simulink model "TST_RmtAPP_Kickdown"  (R2016b)
settings: Solver=FixedStepDiscrete  StartTime=0.0  StopTime=simTime  FixedStep=sampleTime  RelTol=1e-3
values from neighbouring files (symbols this model uses):
  testCase = 1    [initTST_RmtAPP_Kickdown_001.m]    (also in initTST_RmtAPP_Kickdown_002.m = 2; initTST_RmtAPP_Kickdown_003.m = 3)
libraries: simulink x7, UnitTest_Lib x3
settings Model: Creator=bianxuyin  LastModifiedBy=bianxuyin
settings DebuggingCC: SignalRangeChecking=error

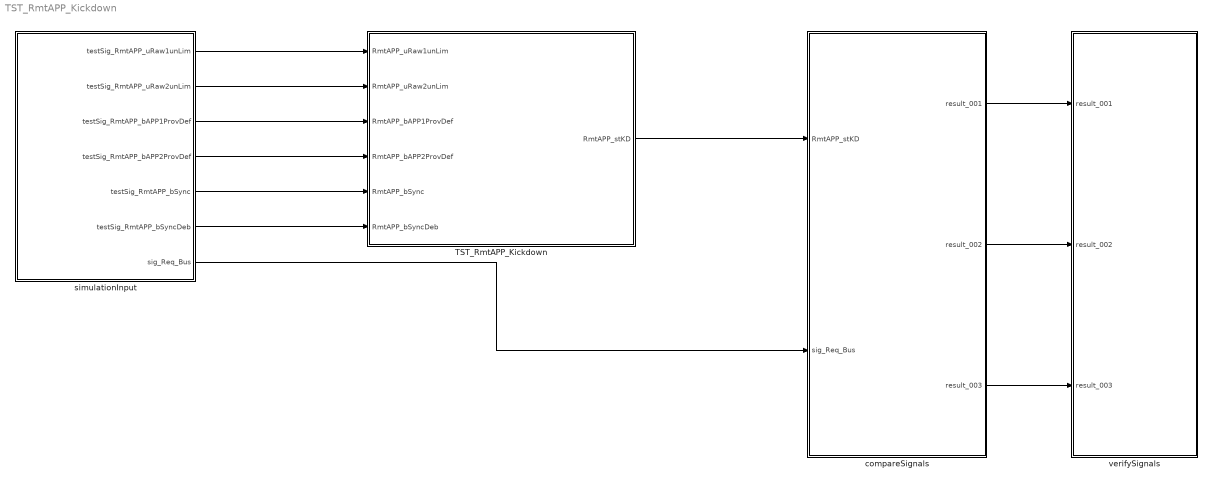
== system TST_RmtAPP_Kickdown ==
  TST_RmtAPP_Kickdown : Subsystem
  compareSignals : Subsystem
  simulationInput : Subsystem
  verifySignals : Subsystem
  wires:
  simulationInput/1(testSig_RmtAPP_uRaw1unLim) -> TST_RmtAPP_Kickdown/1(RmtAPP_uRaw1unLim)
  simulationInput/2(testSig_RmtAPP_uRaw2unLim) -> TST_RmtAPP_Kickdown/2(RmtAPP_uRaw2unLim)
  simulationInput/3(testSig_RmtAPP_bAPP1ProvDef) -> TST_RmtAPP_Kickdown/3(RmtAPP_bAPP1ProvDef)
  simulationInput/4(testSig_RmtAPP_bAPP2ProvDef) -> TST_RmtAPP_Kickdown/4(RmtAPP_bAPP2ProvDef)
  simulationInput/5(testSig_RmtAPP_bSync) -> TST_RmtAPP_Kickdown/5(RmtAPP_bSync)
  simulationInput/6(testSig_RmtAPP_bSyncDeb) -> TST_RmtAPP_Kickdown/6(RmtAPP_bSyncDeb)
  TST_RmtAPP_Kickdown/1(RmtAPP_stKD) -> compareSignals/1(RmtAPP_stKD)
  simulationInput/7(sig_Req_Bus) -> compareSignals/2(sig_Req_Bus)
  compareSignals/1(result_001) -> verifySignals/1(result_001)
  compareSignals/2(result_002) -> verifySignals/2(result_002)
  compareSignals/3(result_003) -> verifySignals/3(result_003)

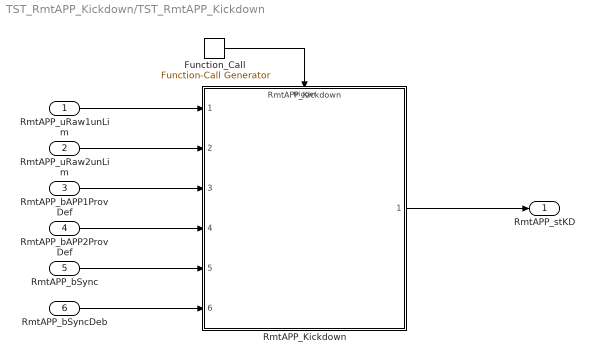
== system TST_RmtAPP_Kickdown/TST_RmtAPP_Kickdown ==
  RmtAPP_uRaw1unLim : Inport
  RmtAPP_uRaw2unLim : Inport  Port=2
  RmtAPP_bAPP1ProvDef : Inport  Port=3
  RmtAPP_bAPP2ProvDef : Inport  Port=4
  RmtAPP_bSync : Inport  Port=5
  RmtAPP_bSyncDeb : Inport  Port=6
  Function_Call : simulink/Ports & Subsystems/Function-Call Generator  sample_time=sampleTime  numberOfIterations=1
  RmtAPP_Kickdown : ModelReference  ModelNameDialog=RmtAPP_Kickdown  SimulationMode=Normal  ModelReferenceVersion=1.3  TriggerPortName=function  TriggerPortTriggerType=function-call  TriggerPortStatesWhenEnabling=held
  RmtAPP_stKD : Outport
  wires:
  Function_Call/1 -> RmtAPP_Kickdown/Trigger
  RmtAPP_uRaw1unLim/1 -> RmtAPP_Kickdown/1
  RmtAPP_uRaw2unLim/1 -> RmtAPP_Kickdown/2
  RmtAPP_bAPP1ProvDef/1 -> RmtAPP_Kickdown/3
  RmtAPP_bAPP2ProvDef/1 -> RmtAPP_Kickdown/4
  RmtAPP_bSync/1 -> RmtAPP_Kickdown/5
  RmtAPP_bSyncDeb/1 -> RmtAPP_Kickdown/6
  RmtAPP_Kickdown/1 -> RmtAPP_stKD/1

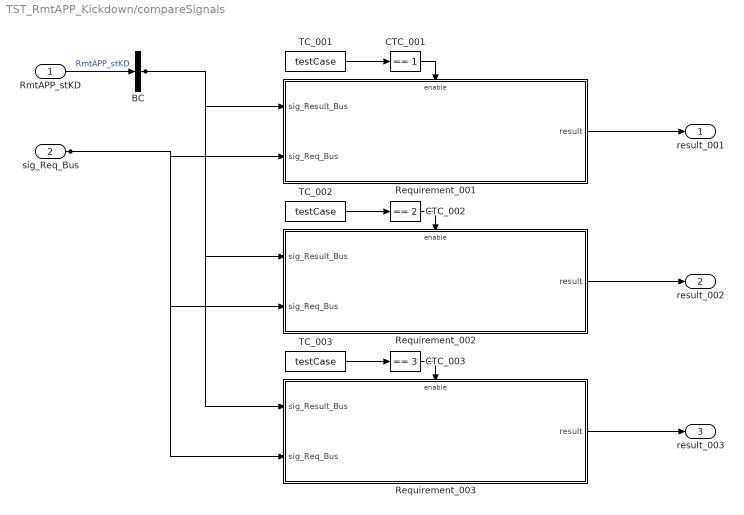
== system TST_RmtAPP_Kickdown/compareSignals ==
  RmtAPP_stKD : Inport
  sig_Req_Bus : Inport  Port=2
  BC : BusCreator  Inputs=1
  CTC_001 : simulink/Logic and Bit Operations/Compare To Constant  relop===  const=1  OutDataTypeStr=boolean
  CTC_002 : simulink/Logic and Bit Operations/Compare To Constant  relop===  const=2  OutDataTypeStr=boolean
  CTC_003 : simulink/Logic and Bit Operations/Compare To Constant  relop===  const=3  OutDataTypeStr=boolean
  Requirement_001 : Subsystem
  Requirement_002 : Subsystem
  Requirement_003 : Subsystem
  TC_001 : Constant  Value=testCase
  TC_002 : Constant  Value=testCase
  TC_003 : Constant  Value=testCase
  result_001 : Outport
  result_002 : Outport  Port=2
  result_003 : Outport  Port=3
  wires:
  RmtAPP_stKD/1 -> BC/1  "RmtAPP_stKD"
  TC_001/1 -> CTC_001/1
  CTC_001/1 -> Requirement_001/Enable
  sig_Req_Bus/1 -> Requirement_001/2(sig_Req_Bus), Requirement_002/2(sig_Req_Bus), Requirement_003/2(sig_Req_Bus)
  BC/1 -> Requirement_001/1(sig_Result_Bus), Requirement_002/1(sig_Result_Bus), Requirement_003/1(sig_Result_Bus)
  Requirement_001/1(result) -> result_001/1
  TC_002/1 -> CTC_002/1
  CTC_002/1 -> Requirement_002/Enable
  Requirement_002/1(result) -> result_002/1
  TC_003/1 -> CTC_003/1
  CTC_003/1 -> Requirement_003/Enable
  Requirement_003/1(result) -> result_003/1

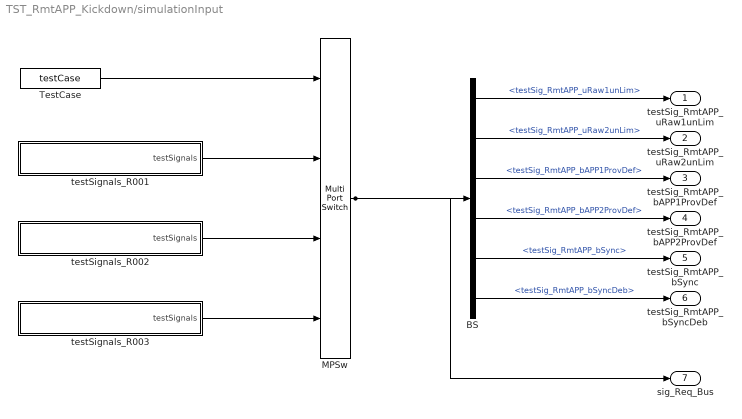
== system TST_RmtAPP_Kickdown/simulationInput ==
  BS : BusSelector  OutputSignals=testSig_RmtAPP_uRaw1unLim,testSig_RmtAPP_uRaw2unLim,testSig_RmtAPP_bAPP1ProvDef,testSig_RmtAPP_bAPP2ProvDef,testSig_RmtAPP_bSync,testSig_RmtAPP_bSyncDeb
  MPSw : MultiPortSwitch  SaturateOnIntegerOverflow=on  InputSameDT=on
  TestCase : Constant  Value=testCase
  testSignals_R001 : Subsystem
  testSignals_R002 : Subsystem
  testSignals_R003 : Subsystem
  testSig_RmtAPP_uRaw1unLim : Outport
  testSig_RmtAPP_uRaw2unLim : Outport  Port=2
  testSig_RmtAPP_bAPP1ProvDef : Outport  Port=3
  testSig_RmtAPP_bAPP2ProvDef : Outport  Port=4
  testSig_RmtAPP_bSync : Outport  Port=5
  testSig_RmtAPP_bSyncDeb : Outport  Port=6
  sig_Req_Bus : Outport  Port=7
  wires:
  BS/1 -> testSig_RmtAPP_uRaw1unLim/1  "<testSig_RmtAPP_uRaw1unLim>"
  BS/2 -> testSig_RmtAPP_uRaw2unLim/1  "<testSig_RmtAPP_uRaw2unLim>"
  BS/3 -> testSig_RmtAPP_bAPP1ProvDef/1  "<testSig_RmtAPP_bAPP1ProvDef>"
  BS/4 -> testSig_RmtAPP_bAPP2ProvDef/1  "<testSig_RmtAPP_bAPP2ProvDef>"
  BS/5 -> testSig_RmtAPP_bSync/1  "<testSig_RmtAPP_bSync>"
  BS/6 -> testSig_RmtAPP_bSyncDeb/1  "<testSig_RmtAPP_bSyncDeb>"
  MPSw/1 -> BS/1, sig_Req_Bus/1
  TestCase/1 -> MPSw/1
  testSignals_R001/1(testSignals) -> MPSw/2
  testSignals_R002/1(testSignals) -> MPSw/3
  testSignals_R003/1(testSignals) -> MPSw/4

== system TST_RmtAPP_Kickdown/verifySignals ==
  result_001 : Inport
  result_002 : Inport  Port=2
  result_003 : Inport  Port=3
  Assertion_001 : Assertion  Enabled=off
  Assertion_002 : Assertion  Enabled=off
  Assertion_003 : Assertion  Enabled=off
  wires:
  result_001/1 -> Assertion_001/1
  result_002/1 -> Assertion_002/1
  result_003/1 -> Assertion_003/1

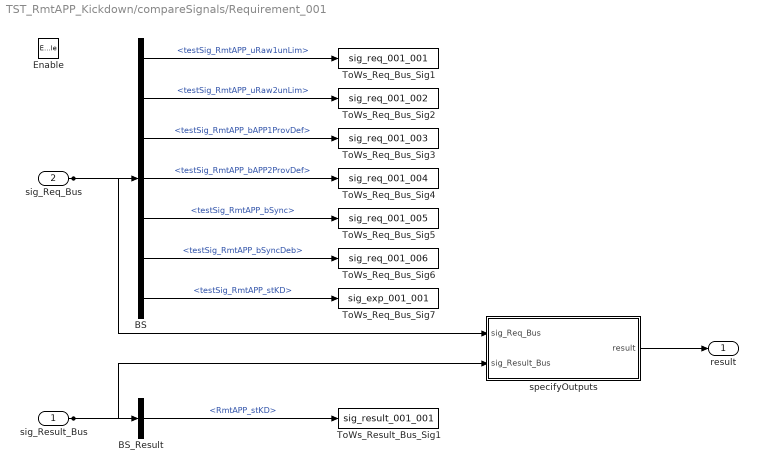
== system TST_RmtAPP_Kickdown/compareSignals/Requirement_001 ==
  sig_Result_Bus : Inport
  sig_Req_Bus : Inport  Port=2
  Enable : EnablePort
  BS : BusSelector  OutputSignals=testSig_RmtAPP_uRaw1unLim,testSig_RmtAPP_uRaw2unLim,testSig_RmtAPP_bAPP1ProvDef,testSig_RmtAPP_bAPP2ProvDef,testSig_RmtAPP_bSync,testSig_RmtAPP_bSyncDeb,testSig_RmtAPP_stKD
  BS_Result : BusSelector  OutputSignals=RmtAPP_stKD
  ToWs_Req_Bus_Sig1 : ToWorkspace  VariableName=sig_req_001_001  SaveFormat=Structure With Time
  ToWs_Req_Bus_Sig2 : ToWorkspace  VariableName=sig_req_001_002  SaveFormat=Structure With Time
  ToWs_Req_Bus_Sig3 : ToWorkspace  VariableName=sig_req_001_003  SaveFormat=Structure With Time
  ToWs_Req_Bus_Sig4 : ToWorkspace  VariableName=sig_req_001_004  SaveFormat=Structure With Time
  ToWs_Req_Bus_Sig5 : ToWorkspace  VariableName=sig_req_001_005  SaveFormat=Structure With Time
  ToWs_Req_Bus_Sig6 : ToWorkspace  VariableName=sig_req_001_006  SaveFormat=Structure With Time
  ToWs_Req_Bus_Sig7 : ToWorkspace  VariableName=sig_exp_001_001  SaveFormat=Structure With Time
  ToWs_Result_Bus_Sig1 : ToWorkspace  VariableName=sig_result_001_001  SaveFormat=Structure With Time
  specifyOutputs : Subsystem
  result : Outport
  wires:
  sig_Req_Bus/1 -> BS/1, specifyOutputs/1(sig_Req_Bus)
  BS/1 -> ToWs_Req_Bus_Sig1/1  "<testSig_RmtAPP_uRaw1unLim>"
  BS/2 -> ToWs_Req_Bus_Sig2/1  "<testSig_RmtAPP_uRaw2unLim>"
  BS/3 -> ToWs_Req_Bus_Sig3/1  "<testSig_RmtAPP_bAPP1ProvDef>"
  BS/4 -> ToWs_Req_Bus_Sig4/1  "<testSig_RmtAPP_bAPP2ProvDef>"
  BS/5 -> ToWs_Req_Bus_Sig5/1  "<testSig_RmtAPP_bSync>"
  BS/6 -> ToWs_Req_Bus_Sig6/1  "<testSig_RmtAPP_bSyncDeb>"
  BS/7 -> ToWs_Req_Bus_Sig7/1  "<testSig_RmtAPP_stKD>"
  sig_Result_Bus/1 -> BS_Result/1, specifyOutputs/2(sig_Result_Bus)
  BS_Result/1 -> ToWs_Result_Bus_Sig1/1  "<RmtAPP_stKD>"
  specifyOutputs/1(result) -> result/1

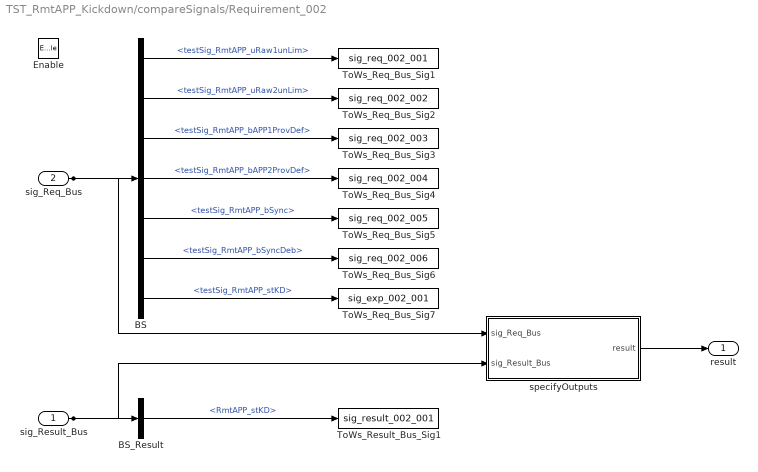
== system TST_RmtAPP_Kickdown/compareSignals/Requirement_002 ==
  sig_Result_Bus : Inport
  sig_Req_Bus : Inport  Port=2
  Enable : EnablePort
  BS : BusSelector  OutputSignals=testSig_RmtAPP_uRaw1unLim,testSig_RmtAPP_uRaw2unLim,testSig_RmtAPP_bAPP1ProvDef,testSig_RmtAPP_bAPP2ProvDef,testSig_RmtAPP_bSync,testSig_RmtAPP_bSyncDeb,testSig_RmtAPP_stKD
  BS_Result : BusSelector  OutputSignals=RmtAPP_stKD
  ToWs_Req_Bus_Sig1 : ToWorkspace  VariableName=sig_req_002_001  SaveFormat=Structure With Time
  ToWs_Req_Bus_Sig2 : ToWorkspace  VariableName=sig_req_002_002  SaveFormat=Structure With Time
  ToWs_Req_Bus_Sig3 : ToWorkspace  VariableName=sig_req_002_003  SaveFormat=Structure With Time
  ToWs_Req_Bus_Sig4 : ToWorkspace  VariableName=sig_req_002_004  SaveFormat=Structure With Time
  ToWs_Req_Bus_Sig5 : ToWorkspace  VariableName=sig_req_002_005  SaveFormat=Structure With Time
  ToWs_Req_Bus_Sig6 : ToWorkspace  VariableName=sig_req_002_006  SaveFormat=Structure With Time
  ToWs_Req_Bus_Sig7 : ToWorkspace  VariableName=sig_exp_002_001  SaveFormat=Structure With Time
  ToWs_Result_Bus_Sig1 : ToWorkspace  VariableName=sig_result_002_001  SaveFormat=Structure With Time
  specifyOutputs : Subsystem
  result : Outport
  wires:
  sig_Req_Bus/1 -> BS/1, specifyOutputs/1(sig_Req_Bus)
  BS/1 -> ToWs_Req_Bus_Sig1/1  "<testSig_RmtAPP_uRaw1unLim>"
  BS/2 -> ToWs_Req_Bus_Sig2/1  "<testSig_RmtAPP_uRaw2unLim>"
  BS/3 -> ToWs_Req_Bus_Sig3/1  "<testSig_RmtAPP_bAPP1ProvDef>"
  BS/4 -> ToWs_Req_Bus_Sig4/1  "<testSig_RmtAPP_bAPP2ProvDef>"
  BS/5 -> ToWs_Req_Bus_Sig5/1  "<testSig_RmtAPP_bSync>"
  BS/6 -> ToWs_Req_Bus_Sig6/1  "<testSig_RmtAPP_bSyncDeb>"
  BS/7 -> ToWs_Req_Bus_Sig7/1  "<testSig_RmtAPP_stKD>"
  sig_Result_Bus/1 -> BS_Result/1, specifyOutputs/2(sig_Result_Bus)
  BS_Result/1 -> ToWs_Result_Bus_Sig1/1  "<RmtAPP_stKD>"
  specifyOutputs/1(result) -> result/1

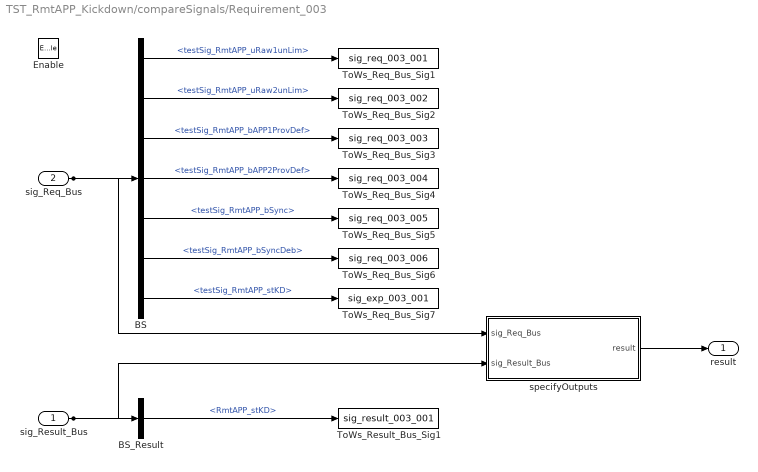
== system TST_RmtAPP_Kickdown/compareSignals/Requirement_003 ==
  sig_Result_Bus : Inport
  sig_Req_Bus : Inport  Port=2
  Enable : EnablePort
  BS : BusSelector  OutputSignals=testSig_RmtAPP_uRaw1unLim,testSig_RmtAPP_uRaw2unLim,testSig_RmtAPP_bAPP1ProvDef,testSig_RmtAPP_bAPP2ProvDef,testSig_RmtAPP_bSync,testSig_RmtAPP_bSyncDeb,testSig_RmtAPP_stKD
  BS_Result : BusSelector  OutputSignals=RmtAPP_stKD
  ToWs_Req_Bus_Sig1 : ToWorkspace  VariableName=sig_req_003_001  SaveFormat=Structure With Time
  ToWs_Req_Bus_Sig2 : ToWorkspace  VariableName=sig_req_003_002  SaveFormat=Structure With Time
  ToWs_Req_Bus_Sig3 : ToWorkspace  VariableName=sig_req_003_003  SaveFormat=Structure With Time
  ToWs_Req_Bus_Sig4 : ToWorkspace  VariableName=sig_req_003_004  SaveFormat=Structure With Time
  ToWs_Req_Bus_Sig5 : ToWorkspace  VariableName=sig_req_003_005  SaveFormat=Structure With Time
  ToWs_Req_Bus_Sig6 : ToWorkspace  VariableName=sig_req_003_006  SaveFormat=Structure With Time
  ToWs_Req_Bus_Sig7 : ToWorkspace  VariableName=sig_exp_003_001  SaveFormat=Structure With Time
  ToWs_Result_Bus_Sig1 : ToWorkspace  VariableName=sig_result_003_001  SaveFormat=Structure With Time
  specifyOutputs : Subsystem
  result : Outport
  wires:
  sig_Req_Bus/1 -> BS/1, specifyOutputs/1(sig_Req_Bus)
  BS/1 -> ToWs_Req_Bus_Sig1/1  "<testSig_RmtAPP_uRaw1unLim>"
  BS/2 -> ToWs_Req_Bus_Sig2/1  "<testSig_RmtAPP_uRaw2unLim>"
  BS/3 -> ToWs_Req_Bus_Sig3/1  "<testSig_RmtAPP_bAPP1ProvDef>"
  BS/4 -> ToWs_Req_Bus_Sig4/1  "<testSig_RmtAPP_bAPP2ProvDef>"
  BS/5 -> ToWs_Req_Bus_Sig5/1  "<testSig_RmtAPP_bSync>"
  BS/6 -> ToWs_Req_Bus_Sig6/1  "<testSig_RmtAPP_bSyncDeb>"
  BS/7 -> ToWs_Req_Bus_Sig7/1  "<testSig_RmtAPP_stKD>"
  sig_Result_Bus/1 -> BS_Result/1, specifyOutputs/2(sig_Result_Bus)
  BS_Result/1 -> ToWs_Result_Bus_Sig1/1  "<RmtAPP_stKD>"
  specifyOutputs/1(result) -> result/1

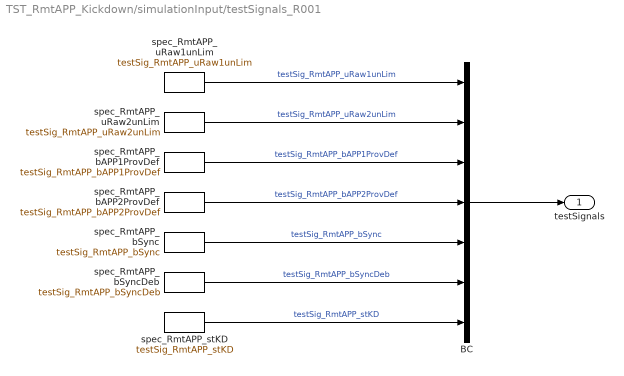
== system TST_RmtAPP_Kickdown/simulationInput/testSignals_R001 ==
  BC : BusCreator  Inputs=7
  spec_RmtAPP_bAPP1ProvDef : FromWorkspace  VariableName=testSig_RmtAPP_bAPP1ProvDef  Interpolate=off  OutputAfterFinalValue=Holding final value
  spec_RmtAPP_bAPP2ProvDef : FromWorkspace  VariableName=testSig_RmtAPP_bAPP2ProvDef  Interpolate=off  OutputAfterFinalValue=Holding final value
  spec_RmtAPP_bSync : FromWorkspace  VariableName=testSig_RmtAPP_bSync  Interpolate=off  OutputAfterFinalValue=Holding final value
  spec_RmtAPP_bSyncDeb : FromWorkspace  VariableName=testSig_RmtAPP_bSyncDeb  Interpolate=off  OutputAfterFinalValue=Holding final value
  spec_RmtAPP_stKD : FromWorkspace  VariableName=testSig_RmtAPP_stKD  Interpolate=off  OutputAfterFinalValue=Holding final value
  spec_RmtAPP_uRaw1unLim : FromWorkspace  VariableName=testSig_RmtAPP_uRaw1unLim  Interpolate=off  OutputAfterFinalValue=Holding final value
  spec_RmtAPP_uRaw2unLim : FromWorkspace  VariableName=testSig_RmtAPP_uRaw2unLim  Interpolate=off  OutputAfterFinalValue=Holding final value
  testSignals : Outport
  wires:
  BC/1 -> testSignals/1
  spec_RmtAPP_uRaw1unLim/1 -> BC/1  "testSig_RmtAPP_uRaw1unLim"
  spec_RmtAPP_uRaw2unLim/1 -> BC/2  "testSig_RmtAPP_uRaw2unLim"
  spec_RmtAPP_bAPP1ProvDef/1 -> BC/3  "testSig_RmtAPP_bAPP1ProvDef"
  spec_RmtAPP_bAPP2ProvDef/1 -> BC/4  "testSig_RmtAPP_bAPP2ProvDef"
  spec_RmtAPP_bSync/1 -> BC/5  "testSig_RmtAPP_bSync"
  spec_RmtAPP_bSyncDeb/1 -> BC/6  "testSig_RmtAPP_bSyncDeb"
  spec_RmtAPP_stKD/1 -> BC/7  "testSig_RmtAPP_stKD"

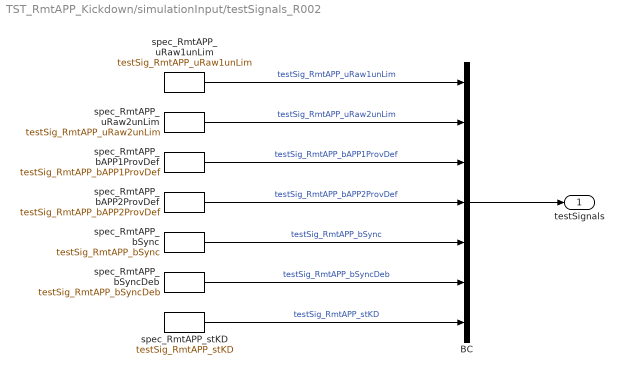
== system TST_RmtAPP_Kickdown/simulationInput/testSignals_R002 ==
  BC : BusCreator  Inputs=7
  spec_RmtAPP_bAPP1ProvDef : FromWorkspace  VariableName=testSig_RmtAPP_bAPP1ProvDef  Interpolate=off  OutputAfterFinalValue=Holding final value
  spec_RmtAPP_bAPP2ProvDef : FromWorkspace  VariableName=testSig_RmtAPP_bAPP2ProvDef  Interpolate=off  OutputAfterFinalValue=Holding final value
  spec_RmtAPP_bSync : FromWorkspace  VariableName=testSig_RmtAPP_bSync  Interpolate=off  OutputAfterFinalValue=Holding final value
  spec_RmtAPP_bSyncDeb : FromWorkspace  VariableName=testSig_RmtAPP_bSyncDeb  Interpolate=off  OutputAfterFinalValue=Holding final value
  spec_RmtAPP_stKD : FromWorkspace  VariableName=testSig_RmtAPP_stKD  Interpolate=off  OutputAfterFinalValue=Holding final value
  spec_RmtAPP_uRaw1unLim : FromWorkspace  VariableName=testSig_RmtAPP_uRaw1unLim  Interpolate=off  OutputAfterFinalValue=Holding final value
  spec_RmtAPP_uRaw2unLim : FromWorkspace  VariableName=testSig_RmtAPP_uRaw2unLim  Interpolate=off  OutputAfterFinalValue=Holding final value
  testSignals : Outport
  wires:
  BC/1 -> testSignals/1
  spec_RmtAPP_uRaw1unLim/1 -> BC/1  "testSig_RmtAPP_uRaw1unLim"
  spec_RmtAPP_uRaw2unLim/1 -> BC/2  "testSig_RmtAPP_uRaw2unLim"
  spec_RmtAPP_bAPP1ProvDef/1 -> BC/3  "testSig_RmtAPP_bAPP1ProvDef"
  spec_RmtAPP_bAPP2ProvDef/1 -> BC/4  "testSig_RmtAPP_bAPP2ProvDef"
  spec_RmtAPP_bSync/1 -> BC/5  "testSig_RmtAPP_bSync"
  spec_RmtAPP_bSyncDeb/1 -> BC/6  "testSig_RmtAPP_bSyncDeb"
  spec_RmtAPP_stKD/1 -> BC/7  "testSig_RmtAPP_stKD"

== system TST_RmtAPP_Kickdown/simulationInput/testSignals_R003 ==
  BC : BusCreator  Inputs=7
  spec_RmtAPP_bAPP1ProvDef : FromWorkspace  VariableName=testSig_RmtAPP_bAPP1ProvDef  Interpolate=off  OutputAfterFinalValue=Holding final value
  spec_RmtAPP_bAPP2ProvDef : FromWorkspace  VariableName=testSig_RmtAPP_bAPP2ProvDef  Interpolate=off  OutputAfterFinalValue=Holding final value
  spec_RmtAPP_bSync : FromWorkspace  VariableName=testSig_RmtAPP_bSync  Interpolate=off  OutputAfterFinalValue=Holding final value
  spec_RmtAPP_bSyncDeb : FromWorkspace  VariableName=testSig_RmtAPP_bSyncDeb  Interpolate=off  OutputAfterFinalValue=Holding final value
  spec_RmtAPP_stKD : FromWorkspace  VariableName=testSig_RmtAPP_stKD  Interpolate=off  OutputAfterFinalValue=Holding final value
  spec_RmtAPP_uRaw1unLim : FromWorkspace  VariableName=testSig_RmtAPP_uRaw1unLim  Interpolate=off  OutputAfterFinalValue=Holding final value
  spec_RmtAPP_uRaw2unLim : FromWorkspace  VariableName=testSig_RmtAPP_uRaw2unLim  Interpolate=off  OutputAfterFinalValue=Holding final value
  testSignals : Outport
  wires:
  BC/1 -> testSignals/1
  spec_RmtAPP_uRaw1unLim/1 -> BC/1  "testSig_RmtAPP_uRaw1unLim"
  spec_RmtAPP_uRaw2unLim/1 -> BC/2  "testSig_RmtAPP_uRaw2unLim"
  spec_RmtAPP_bAPP1ProvDef/1 -> BC/3  "testSig_RmtAPP_bAPP1ProvDef"
  spec_RmtAPP_bAPP2ProvDef/1 -> BC/4  "testSig_RmtAPP_bAPP2ProvDef"
  spec_RmtAPP_bSync/1 -> BC/5  "testSig_RmtAPP_bSync"
  spec_RmtAPP_bSyncDeb/1 -> BC/6  "testSig_RmtAPP_bSyncDeb"
  spec_RmtAPP_stKD/1 -> BC/7  "testSig_RmtAPP_stKD"

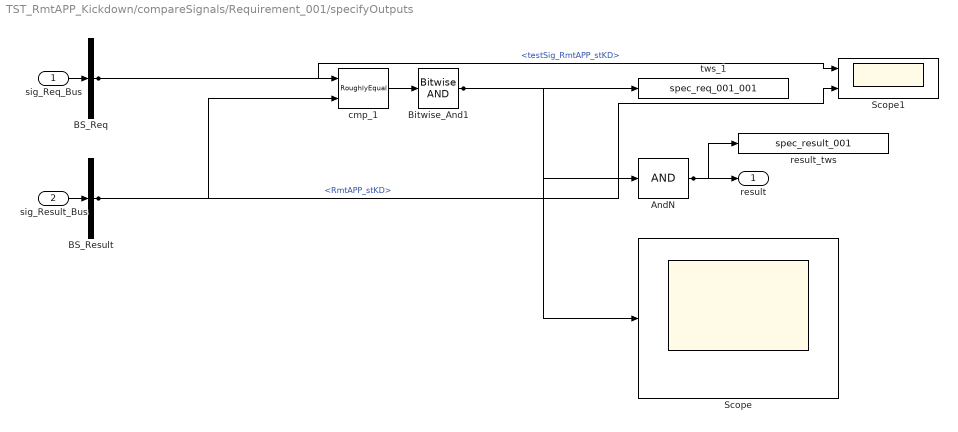
== system TST_RmtAPP_Kickdown/compareSignals/Requirement_001/specifyOutputs ==
  sig_Req_Bus : Inport
  sig_Result_Bus : Inport  Port=2
  AndN : Logic  Inputs=1
  BS_Req : BusSelector  OutputSignals=testSig_RmtAPP_stKD
  BS_Result : BusSelector  OutputSignals=RmtAPP_stKD
  Bitwise_And1 : simulink/Logic and Bit Operations/Bitwise Operator  logicop=AND  UseBitMask=off  BitMask=bin2dec('11011001')  BitMaskRealWorld=Stored Integer
  Scope : Scope
  Scope1 : Scope  NumInputPorts=2
  cmp_1 : UnitTest_Lib/RoughlyEqual  slope=0.1
  result_tws : ToWorkspace  VariableName=spec_result_001
  tws_1 : ToWorkspace  VariableName=spec_req_001_001
  result : Outport
  wires:
  sig_Req_Bus/1 -> BS_Req/1
  sig_Result_Bus/1 -> BS_Result/1
  AndN/1 -> result/1, result_tws/1
  BS_Req/1 -> cmp_1/1, Scope1/1  "<testSig_RmtAPP_stKD>"
  BS_Result/1 -> cmp_1/2, Scope1/2  "<RmtAPP_stKD>"
  cmp_1/1 -> Bitwise_And1/1
  Bitwise_And1/1 -> tws_1/1, AndN/1, Scope/1

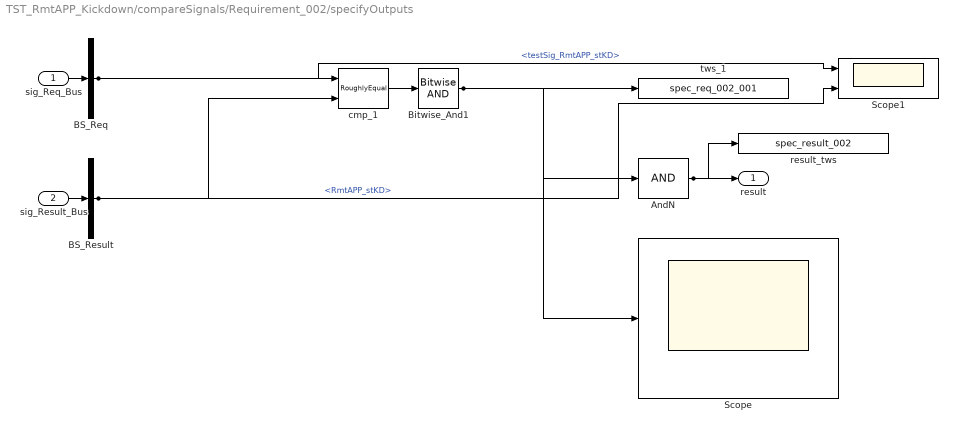
== system TST_RmtAPP_Kickdown/compareSignals/Requirement_002/specifyOutputs ==
  sig_Req_Bus : Inport
  sig_Result_Bus : Inport  Port=2
  AndN : Logic  Inputs=1
  BS_Req : BusSelector  OutputSignals=testSig_RmtAPP_stKD
  BS_Result : BusSelector  OutputSignals=RmtAPP_stKD
  Bitwise_And1 : simulink/Logic and Bit Operations/Bitwise Operator  logicop=AND  UseBitMask=off  BitMask=bin2dec('11011001')  BitMaskRealWorld=Stored Integer
  Scope : Scope
  Scope1 : Scope  NumInputPorts=2
  cmp_1 : UnitTest_Lib/RoughlyEqual  slope=0.1
  result_tws : ToWorkspace  VariableName=spec_result_002
  tws_1 : ToWorkspace  VariableName=spec_req_002_001
  result : Outport
  wires:
  sig_Req_Bus/1 -> BS_Req/1
  sig_Result_Bus/1 -> BS_Result/1
  AndN/1 -> result/1, result_tws/1
  BS_Req/1 -> cmp_1/1, Scope1/1  "<testSig_RmtAPP_stKD>"
  BS_Result/1 -> cmp_1/2, Scope1/2  "<RmtAPP_stKD>"
  cmp_1/1 -> Bitwise_And1/1
  Bitwise_And1/1 -> tws_1/1, AndN/1, Scope/1

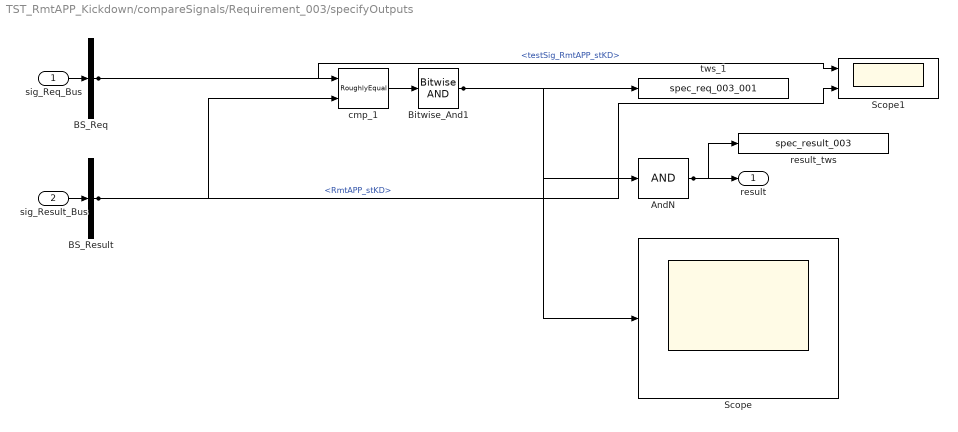
== system TST_RmtAPP_Kickdown/compareSignals/Requirement_003/specifyOutputs ==
  sig_Req_Bus : Inport
  sig_Result_Bus : Inport  Port=2
  AndN : Logic  Inputs=1
  BS_Req : BusSelector  OutputSignals=testSig_RmtAPP_stKD
  BS_Result : BusSelector  OutputSignals=RmtAPP_stKD
  Bitwise_And1 : simulink/Logic and Bit Operations/Bitwise Operator  logicop=AND  UseBitMask=off  BitMask=bin2dec('11011001')  BitMaskRealWorld=Stored Integer
  Scope : Scope
  Scope1 : Scope  NumInputPorts=2
  cmp_1 : UnitTest_Lib/RoughlyEqual  slope=0.1
  result_tws : ToWorkspace  VariableName=spec_result_003
  tws_1 : ToWorkspace  VariableName=spec_req_003_001
  result : Outport
  wires:
  sig_Req_Bus/1 -> BS_Req/1
  sig_Result_Bus/1 -> BS_Result/1
  AndN/1 -> result/1, result_tws/1
  BS_Req/1 -> cmp_1/1, Scope1/1  "<testSig_RmtAPP_stKD>"
  BS_Result/1 -> cmp_1/2, Scope1/2  "<RmtAPP_stKD>"
  cmp_1/1 -> Bitwise_And1/1
  Bitwise_And1/1 -> tws_1/1, AndN/1, Scope/1
